simulink model "tracknshoot"  (R2017a)
settings: Solver=FixedStepDiscrete  StartTime=0.0  StopTime=10.0  FixedStep=0.001  RelTol=1e-3
libraries: stellaris_lp_lib x17, simulink x3, etargetslib x1, commutil2 x1, xpcutilitieslib x1
settings Model: ExtModeTrigDuration=8  Creator=peselnikmg  LastModifiedBy=Stewart
settings DataIOCC: LimitDataPoints=on  SaveFormat=Array  SignalLoggingSaveFormat=ModelDataLogs  ReturnWorkspaceOutputs=on
settings OptimizationCC: UseDivisionForNetSlopeComputation=on  UseFloatMulNetSlope=on  DefaultUnderspecifiedDataType=single  UseSpecifiedMinMax=on  PassReuseOutputArgsAs=Individual arguments  ExpressionDepthLimit=2147483647  ZeroExternalMemoryAtStartup=off  NoFixptDivByZeroProtection=on  EfficientFloat2IntCast=on  LifeSpan=inf  MaxStackSize=64  OptimizeBlockOrder=speed
settings DebuggingCC: ReadBeforeWriteMsg=DisableAll  WriteAfterWriteMsg=DisableAll  WriteAfterReadMsg=DisableAll  MultiTaskDSMMsg=none  IntegerOverflowMsg=error  ParameterTunabilityLossMsg=error  AssertControl=DisableAll  StateNameClashWarn=warning  NonBusSignalsTreatedAsBus=error  SFInvalidInputDataAccessInChartInitDiag=error  SFTransitionOutsideNaturalParentDiag=error  SFUnreachableExecutionPathDiag=error  SFUndirectedBroadcastEventsDiag=error  SFExecutionAtInitializationDiag=none  IntegerSaturationMsg=error
settings HardwareCC: ProdBitPerPointer=32  ProdBitPerSizeT=32  ProdBitPerPtrDiffT=32  ProdLargestAtomicInteger=Long  ProdLargestAtomicFloat=Double  ProdWordSize=32  ProdHWDeviceType=ARM Compatible->ARM Cortex
settings ModelReferenceCC: UpdateModelReferenceTargets=IfOutOfDate  PropagateSignalLabelsOutOfModel=off
settings SFSimCC: SFSimEcho=off  MATLABDynamicMemAlloc=off
settings RTWCC: SystemTargetFile=ert.tlc  HardwareBoard=Tiva TM4C123G Launchpad  TLCOptions=-aInlineSetEventsForThisBaseRateFcn=TLC_FALSE -aSuppressMultiTaskScheduler=TLC_FALSE -aRateBasedStepFcn=1  TemplateMakefile=ert_default_tmf  Description=Embedded Coder  GenerateReport=on  RTWVerbose=off  Toolchain=Texas Instruments Code Composer Studio (Tiva)  IncludeHyperlinkInReport=on  LaunchReport=on  GenerateTraceInfo=on  GenerateTraceReport=on  GenerateTraceReportSl=on  GenerateTraceReportSf=on  GenerateTraceReportEml=on
settings CodeAppCC: ForceParamTrailComments=on  IgnoreCustomStorageClasses=off  OperatorAnnotations=on  SimulinkDataObjDesc=on  SFDataObjDesc=on  MATLABFcnDesc=on  CustomSymbolStrType=$N$R$M  InsertBlockDesc=on  MATLABSourceComments=on  EnableCustomComments=on  ReqsInCode=on
settings ERTTargetCC: UtilityFuncGeneration=Shared location  CombineSignalStateStructs=on  SuppressErrorStatus=on  SupportNonFinite=off  ParenthesesLevel=Maximum  CastingMode=Standards  EnableSignedLeftShifts=off  EnableSignedRightShifts=off
settings ConfigComp: CovMetricSettings=dw  CovHtmlReporting=on  CovSaveCumulativeToWorkspaceVar=on  CovSaveSingleToWorkspaceVar=on  CovExternalEMLEnable=off

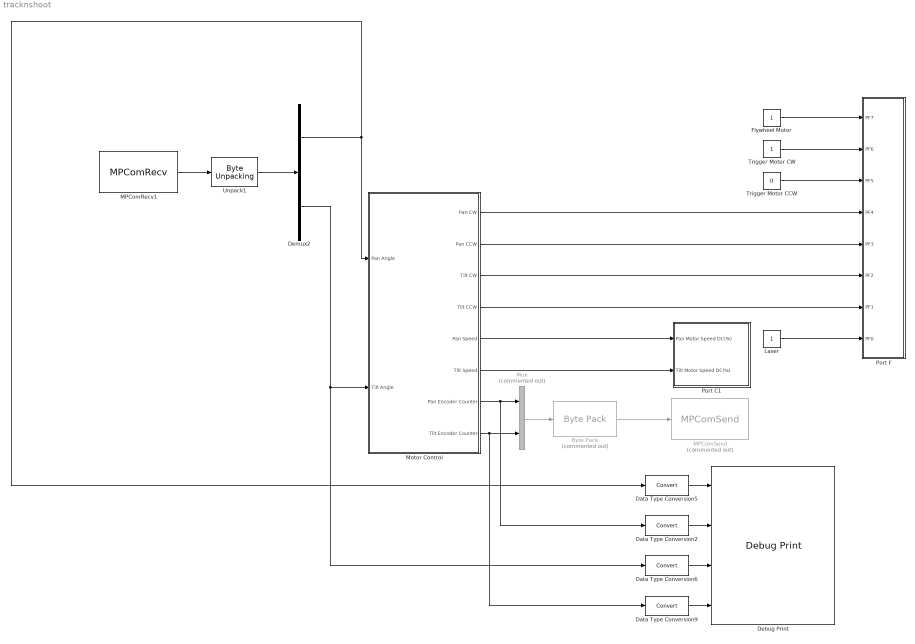
== system tracknshoot ==
  Byte Pack : etargetslib/Byte Pack  Commented=on  datatypes={'double'}  byteAlign=1
  Data Type Conversion{2,5..6,9} (4 alike) : DataTypeConversion
  Debug Print : stellaris_lp_lib/Debug/Debug Print  fmt="'pan: %d %d         tilt: %d %d'"  sample_time=-1
      settings: SourceProductName=Run on Stellaris LaunchPad
  Demux2 : Demux  Outputs=2
  Flywheel Motor : Constant  OutDataTypeStr=uint8
  Laser : Constant  OutDataTypeStr=uint8
  MPComRecv1 : stellaris_lp_lib/Communication/MPComRecv  vport=2  pack_size=8  sample_time=-1
      settings: SourceProductName=Run on Stellaris LaunchPad
  MPComSend : stellaris_lp_lib/Communication/MPComSend  Commented=on  vport=2  pack_size=4  sample_time=0.2
      settings: SourceProductName=Run on Stellaris LaunchPad
  Motor Control : Subsystem
  Mux : Mux  Commented=on  Inputs=2
  Port C1 : Subsystem  TreatAsAtomicUnit=on
  Port F : Subsystem  TreatAsAtomicUnit=on
  Trigger Motor CCW : Constant  Value=0  OutDataTypeStr=uint8
  Trigger Motor CW : Constant  OutDataTypeStr=uint8
  Unpack1 : xpcutilitieslib/Byte Unpacking   MaskUnpackedDataTypes={['single']}  MaskUnpackedDataSizes={[1, 2]}  MaskAlignment=1
      settings: SourceProductName=Simulink Real-Time  SourceProductBaseCode=XP
  wires:
  Trigger Motor CW/1 -> Port F/2(PF6)
  Trigger Motor CCW/1 -> Port F/3(PF5)
  Laser/1 -> Port F/8(PF0)
  Unpack1/1 -> Demux2/1
  MPComRecv1/1 -> Unpack1/1
  Motor Control/1(Pan CW) -> Port F/4(PF4)
  Motor Control/2(Pan CCW) -> Port F/5(PF3)
  Motor Control/3(Tilt CW) -> Port F/6(PF2)
  Motor Control/4(Tilt CCW) -> Port F/7(PF1)
  Motor Control/5(Pan Speed) -> Port C1/1("Pan Motor Speed DC(%) ")
  Motor Control/6(Tilt Speed) -> Port C1/2(Tilt Motor Speed DC(%))
  Data Type Conversion9/1 -> Debug Print/4
  Data Type Conversion2/1 -> Debug Print/2
  Data Type Conversion6/1 -> Debug Print/3
  Data Type Conversion5/1 -> Debug Print/1
  Flywheel Motor/1 -> Port F/1(PF7)
  Mux/1 -> Byte Pack/1
  Byte Pack/1 -> MPComSend/1
  Demux2/1 -> Motor Control/1(Pan Angle), Data Type Conversion5/1
  Demux2/2 -> Data Type Conversion6/1, Motor Control/2(Tilt Angle)
  Motor Control/8(Tilt Encoder Counter) -> Data Type Conversion9/1, Mux/2
  Motor Control/7(Pan Encoder Counter) -> Data Type Conversion2/1, Mux/1

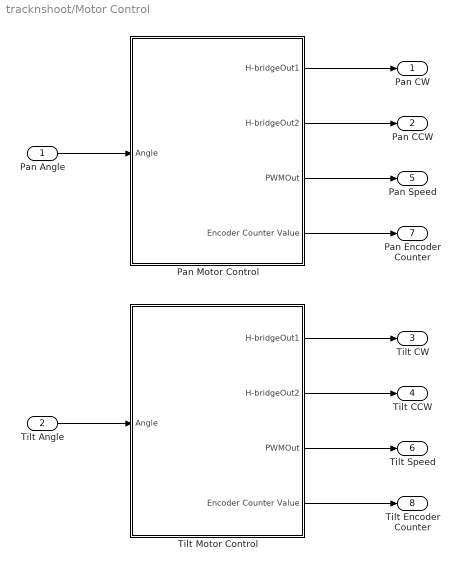
== system tracknshoot/Motor Control ==
  Pan Angle : Inport
  Tilt Angle : Inport  Port=2
  Pan Motor Control : Subsystem
  Tilt Motor Control : Subsystem
  Pan CW : Outport
  Pan CCW : Outport  Port=2
  Tilt CW : Outport  Port=3
  Tilt CCW : Outport  Port=4
  Pan Speed : Outport  Port=5
  Tilt Speed : Outport  Port=6
  Pan Encoder Counter : Outport  Port=7
  Tilt Encoder Counter : Outport  Port=8
  wires:
  Pan Angle/1 -> Pan Motor Control/1(Angle)
  Pan Motor Control/2(H-bridgeOut2) -> Pan CCW/1
  Pan Motor Control/1(H-bridgeOut1) -> Pan CW/1
  Pan Motor Control/4(Encoder Counter Value) -> Pan Encoder Counter/1
  Pan Motor Control/3(PWMOut) -> Pan Speed/1
  Tilt Motor Control/2(H-bridgeOut2) -> Tilt CCW/1
  Tilt Motor Control/3(PWMOut) -> Tilt Speed/1
  Tilt Motor Control/1(H-bridgeOut1) -> Tilt CW/1
  Tilt Motor Control/4(Encoder Counter Value) -> Tilt Encoder Counter/1
  Tilt Angle/1 -> Tilt Motor Control/1(Angle)

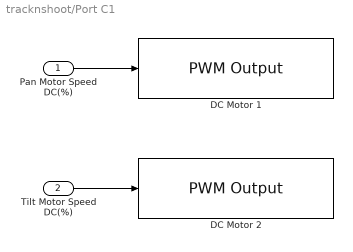
== system tracknshoot/Port C1 ==
  "Pan Motor Speed DC(%) " : Inport  OutDataTypeStr=single
  Tilt Motor Speed DC(%) : Inport  Port=2  OutDataTypeStr=single
  DC Motor 1 : stellaris_lp_lib/PWM/PWM Output  ch="2    PC5"  invert=off  freq=2e4  sample_time=-1
      settings: SourceProductName=Run on Stellaris LaunchPad
  DC Motor 2 : stellaris_lp_lib/PWM/PWM Output  ch="1    PC4"  invert=off  freq=2e4  sample_time=-1
      settings: SourceProductName=Run on Stellaris LaunchPad
  wires:
  "Pan Motor Speed DC(%) "/1 -> DC Motor 1/1
  Tilt Motor Speed DC(%)/1 -> DC Motor 2/1

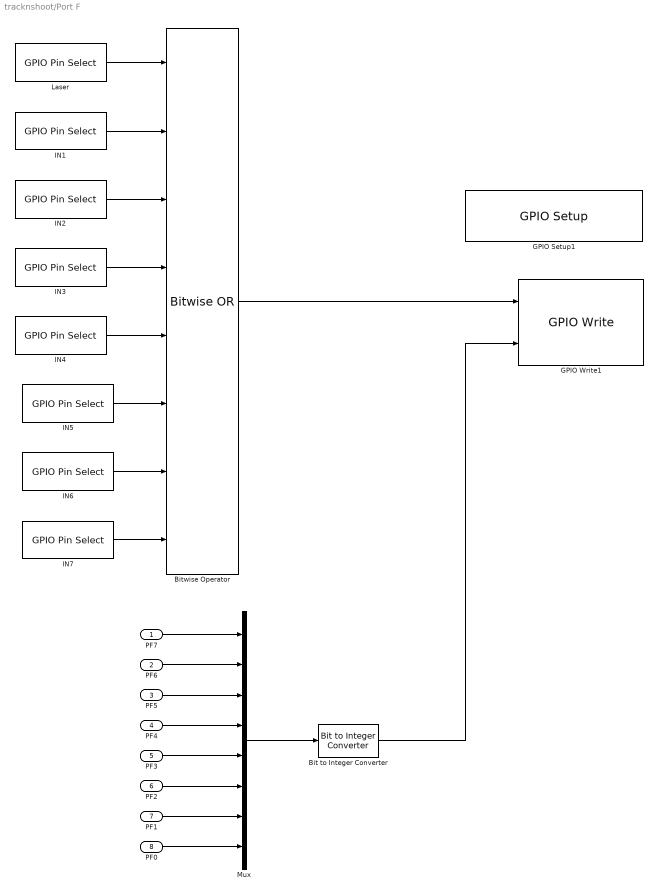
== system tracknshoot/Port F ==
  PF7 : Inport
  PF6 : Inport  Port=2
  PF5 : Inport  Port=3
  PF4 : Inport  Port=4
  PF3 : Inport  Port=5
  PF2 : Inport  Port=6
  PF1 : Inport  Port=7
  PF0 : Inport  Port=8
  Bit to Integer Converter : commutil2/Bit to Integer Converter  nbits=8  bitOrder=MSB first  signedOutputValues=Unsigned  outDtype=Inherit via internal rule  outDtypeSigned=Inherit via internal rule
  Bitwise Operator : simulink/Logic and Bit Operations/Bitwise Operator  logicop=OR  UseBitMask=off  NumInputPorts=8  BitMask=bin2dec('11011001')  BitMaskRealWorld=Stored Integer
  GPIO Setup1 : stellaris_lp_lib/GPIO/GPIO Setup  GPIO_PORTX_BASE=GPIO_PORTF_BASE  PinsOutput_0=Output  PinsOutput_1=Output  PinsOutput_2=Output  PinsOutput_3=Output  PinsOutput_4=Output  PinsOutput_5=Output  PinsOutput_6=Output  PinsOutput_7=Output
      settings: SourceProductName=Run on Stellaris LaunchPad
  GPIO Write1 : stellaris_lp_lib/GPIO/GPIO Write  GPIO_PORTX_BASE=GPIO_PORTF_BASE  SampleTime=-1
      settings: SourceProductName=Run on Stellaris LaunchPad
  IN1 : stellaris_lp_lib/GPIO/GPIO Pin Select  GPIO_PIN_X=GPIO_PIN_1
      settings: SourceProductName=Run on Stellaris LaunchPad
  IN2 : stellaris_lp_lib/GPIO/GPIO Pin Select  GPIO_PIN_X=GPIO_PIN_2
      settings: SourceProductName=Run on Stellaris LaunchPad
  IN3 : stellaris_lp_lib/GPIO/GPIO Pin Select  GPIO_PIN_X=GPIO_PIN_3
      settings: SourceProductName=Run on Stellaris LaunchPad
  IN4 : stellaris_lp_lib/GPIO/GPIO Pin Select  GPIO_PIN_X=GPIO_PIN_4
      settings: SourceProductName=Run on Stellaris LaunchPad
  IN5 : stellaris_lp_lib/GPIO/GPIO Pin Select  GPIO_PIN_X=GPIO_PIN_5
      settings: SourceProductName=Run on Stellaris LaunchPad
  IN6 : stellaris_lp_lib/GPIO/GPIO Pin Select  GPIO_PIN_X=GPIO_PIN_6
      settings: SourceProductName=Run on Stellaris LaunchPad
  IN7 : stellaris_lp_lib/GPIO/GPIO Pin Select  GPIO_PIN_X=GPIO_PIN_7
      settings: SourceProductName=Run on Stellaris LaunchPad
  Laser : stellaris_lp_lib/GPIO/GPIO Pin Select  GPIO_PIN_X=GPIO_PIN_0
      settings: SourceProductName=Run on Stellaris LaunchPad
  Mux : Mux  Inputs=8
  wires:
  IN4/1 -> Bitwise Operator/5
  IN3/1 -> Bitwise Operator/4
  IN6/1 -> Bitwise Operator/7
  IN1/1 -> Bitwise Operator/2
  IN2/1 -> Bitwise Operator/3
  Bitwise Operator/1 -> GPIO Write1/1
  Laser/1 -> Bitwise Operator/1
  IN5/1 -> Bitwise Operator/6
  Mux/1 -> Bit to Integer Converter/1
  Bit to Integer Converter/1 -> GPIO Write1/2
  IN7/1 -> Bitwise Operator/8
  PF0/1 -> Mux/8
  PF1/1 -> Mux/7
  PF2/1 -> Mux/6
  PF3/1 -> Mux/5
  PF4/1 -> Mux/4
  PF5/1 -> Mux/3
  PF6/1 -> Mux/2
  PF7/1 -> Mux/1

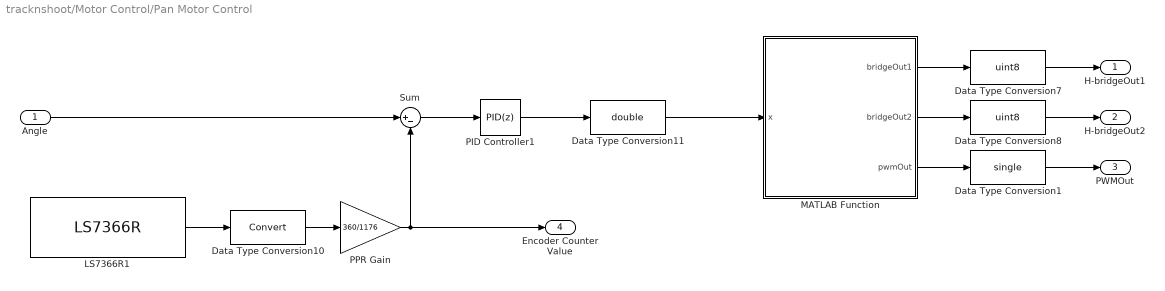
== system tracknshoot/Motor Control/Pan Motor Control ==
  Angle : Inport
  Data Type Conversion1 : DataTypeConversion  OutDataTypeStr=single
  Data Type Conversion10 : DataTypeConversion
  Data Type Conversion11 : DataTypeConversion  OutDataTypeStr=double
  Data Type Conversion7 : DataTypeConversion  OutDataTypeStr=uint8
  Data Type Conversion8 : DataTypeConversion  OutDataTypeStr=uint8
  LS7366R1 : stellaris_lp_lib/SPIDev/LS7366R  ssel="CH 2  (SSEL: PD0)"  ext_clk=on  sample_time=-1
      settings: SourceProductName=Run on Stellaris LaunchPad
  MATLAB Function : MATLAB Function  TreatAsAtomicUnit=on
  PID Controller1 : simulink/Continuous/PID Controller  Controller=PID  TimeDomain=Discrete-time  SampleTime=-1  IntegratorMethod=Forward Euler  FilterMethod=Forward Euler  Form=Parallel  UseFilter=on  ControllerParametersSource=internal  P=2  I=0  D=.05  N=100  InitialConditionSource=internal  InitialConditionForIntegrator=0  InitialConditionForFilter=0  ExternalReset=none  LimitOutput=on  UpperSaturationLimit=50  LowerSaturationLimit=-50  LinearizeAsGain=on  AntiWindupMode=none  Kb=1  TrackingMode=off  Kt=1  PParamMin=[]  PParamMax=[]  IParamMin=[]  IParamMax=[]  DParamMin=[]  DParamMax=[]  NParamMin=[]  NParamMax=[]  KbParamMin=[]  KbParamMax=[]  KtParamMin=[]  KtParamMax=[]  POutMin=[]  POutMax=[]  IOutMin=[]  IOutMax=[]  DOutMin=[]  DOutMax=[]  NOutMin=[]  NOutMax=[]  KbOutMin=[]  KbOutMax=[]  KtOutMin=[]  KtOutMax=[]  IntegratorOutMin=[]  IntegratorOutMax=[]  FilterOutMin=[]  FilterOutMax=[]  SumOutMin=[]  SumOutMax=[]  SumI1OutMin=[]  SumI1OutMax=[]  SumI2OutMin=[]  SumI2OutMax=[]  SumI3OutMin=[]  SumI3OutMax=[]  SumDOutMin=[]  SumDOutMax=[]  SaturationOutMin=[]  SaturationOutMax=[]  IntegratorContinuousStateAttributes=''  IntegratorStateMustResolveToSignalObject=off  IntegratorRTWStateStorageClass=Auto  FilterContinuousStateAttributes=''  FilterStateMustResolveToSignalObject=off  FilterRTWStateStorageClass=Auto  DifferentiatorICPrevScaledInput=0  DifferentiatorOutMin=[]  DifferentiatorOutMax=[]  InitialConditionSetting=State (most efficient)
  PPR Gain : Gain  Gain=360/1176
  Sum : Sum  Inputs=|+-
  H-bridgeOut1 : Outport
  H-bridgeOut2 : Outport  Port=2
  PWMOut : Outport  Port=3
  Encoder Counter Value : Outport  Port=4
  wires:
  LS7366R1/1 -> Data Type Conversion10/1
  PID Controller1/1 -> Data Type Conversion11/1
  Data Type Conversion11/1 -> MATLAB Function/1(x)
  Data Type Conversion10/1 -> PPR Gain/1
  Sum/1 -> PID Controller1/1
  MATLAB Function/1(bridgeOut1) -> Data Type Conversion7/1
  MATLAB Function/2(bridgeOut2) -> Data Type Conversion8/1
  Data Type Conversion8/1 -> H-bridgeOut2/1
  Data Type Conversion7/1 -> H-bridgeOut1/1
  Angle/1 -> Sum/1
  Data Type Conversion1/1 -> PWMOut/1
  MATLAB Function/3(pwmOut) -> Data Type Conversion1/1
  PPR Gain/1 -> Encoder Counter Value/1, Sum/2

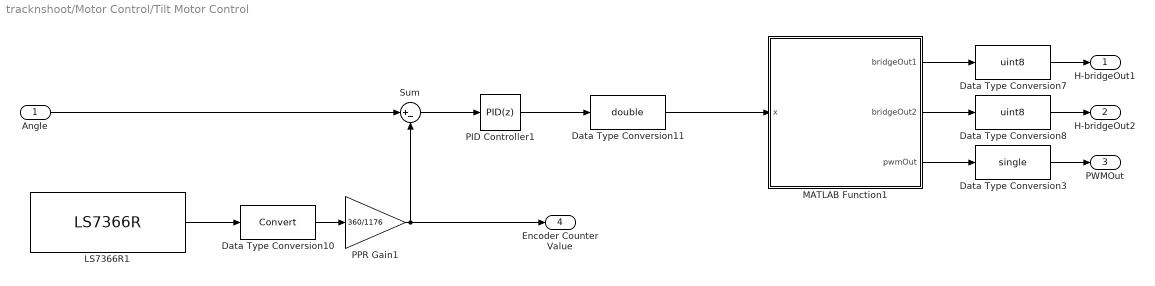
== system tracknshoot/Motor Control/Tilt Motor Control ==
  Angle : Inport
  Data Type Conversion10 : DataTypeConversion
  Data Type Conversion11 : DataTypeConversion  OutDataTypeStr=double
  Data Type Conversion3 : DataTypeConversion  OutDataTypeStr=single
  Data Type Conversion7 : DataTypeConversion  OutDataTypeStr=uint8
  Data Type Conversion8 : DataTypeConversion  OutDataTypeStr=uint8
  LS7366R1 : stellaris_lp_lib/SPIDev/LS7366R  ssel="CH 1  (SSEL: PA3)"  ext_clk=on  sample_time=-1
      settings: SourceProductName=Run on Stellaris LaunchPad
  MATLAB Function1 : MATLAB Function  TreatAsAtomicUnit=on
  PID Controller1 : simulink/Continuous/PID Controller  Controller=PID  TimeDomain=Discrete-time  SampleTime=-1  IntegratorMethod=Forward Euler  FilterMethod=Forward Euler  Form=Parallel  UseFilter=on  ControllerParametersSource=internal  P=2  I=0  D=.05  N=100  InitialConditionSource=internal  InitialConditionForIntegrator=0  InitialConditionForFilter=0  ExternalReset=none  LimitOutput=on  UpperSaturationLimit=25  LowerSaturationLimit=-25  LinearizeAsGain=on  AntiWindupMode=none  Kb=1  TrackingMode=off  Kt=1  PParamMin=[]  PParamMax=[]  IParamMin=[]  IParamMax=[]  DParamMin=[]  DParamMax=[]  NParamMin=[]  NParamMax=[]  KbParamMin=[]  KbParamMax=[]  KtParamMin=[]  KtParamMax=[]  POutMin=[]  POutMax=[]  IOutMin=[]  IOutMax=[]  DOutMin=[]  DOutMax=[]  NOutMin=[]  NOutMax=[]  KbOutMin=[]  KbOutMax=[]  KtOutMin=[]  KtOutMax=[]  IntegratorOutMin=[]  IntegratorOutMax=[]  FilterOutMin=[]  FilterOutMax=[]  SumOutMin=[]  SumOutMax=[]  SumI1OutMin=[]  SumI1OutMax=[]  SumI2OutMin=[]  SumI2OutMax=[]  SumI3OutMin=[]  SumI3OutMax=[]  SumDOutMin=[]  SumDOutMax=[]  SaturationOutMin=[]  SaturationOutMax=[]  IntegratorContinuousStateAttributes=''  IntegratorStateMustResolveToSignalObject=off  IntegratorRTWStateStorageClass=Auto  FilterContinuousStateAttributes=''  FilterStateMustResolveToSignalObject=off  FilterRTWStateStorageClass=Auto  DifferentiatorICPrevScaledInput=0  DifferentiatorOutMin=[]  DifferentiatorOutMax=[]  InitialConditionSetting=State (most efficient)
  PPR Gain1 : Gain  Gain=360/1176
  Sum : Sum  Inputs=|+-
  H-bridgeOut1 : Outport
  H-bridgeOut2 : Outport  Port=2
  PWMOut : Outport  Port=3
  Encoder Counter Value : Outport  Port=4
  wires:
  LS7366R1/1 -> Data Type Conversion10/1
  PID Controller1/1 -> Data Type Conversion11/1
  Data Type Conversion11/1 -> MATLAB Function1/1(x)
  Data Type Conversion10/1 -> PPR Gain1/1
  Sum/1 -> PID Controller1/1
  MATLAB Function1/1(bridgeOut1) -> Data Type Conversion7/1
  MATLAB Function1/2(bridgeOut2) -> Data Type Conversion8/1
  MATLAB Function1/3(pwmOut) -> Data Type Conversion3/1
  Data Type Conversion7/1 -> H-bridgeOut1/1
  Data Type Conversion8/1 -> H-bridgeOut2/1
  Data Type Conversion3/1 -> PWMOut/1
  Angle/1 -> Sum/1
  PPR Gain1/1 -> Encoder Counter Value/1, Sum/2

== matlab function tracknshoot/Motor Control/Tilt Motor Control/MATLAB Function1 ==
  data: bridgeOut1 output; bridgeOut2 output; pwmOut output; x input
function [bridgeOut1, bridgeOut2, pwmOut]= fcn(x)

if x < 0
    bridgeOut1 = 0;
    bridgeOut2 = 1;
    x = -x;
else
    bridgeOut1 = 1;
    bridgeOut2 = 0;
end

pwmOut = x;

== matlab function tracknshoot/Motor Control/Pan Motor Control/MATLAB Function ==
  data: bridgeOut1 output; bridgeOut2 output; pwmOut output; x input
function [bridgeOut1, bridgeOut2, pwmOut]= fcn(x)

if x < 0
    bridgeOut1 = 0;
    bridgeOut2 = 1;
    x = -x;
else
    bridgeOut1 = 1;
    bridgeOut2 = 0;
end

pwmOut = x;
